simulink model "AER372_lab1"  (R2021b)
settings: Solver=VariableStepAuto  StartTime=0.0  StopTime=10.0  RelTol=1e-3
settings Model: Creator=Emma  LastModifiedBy=Emma

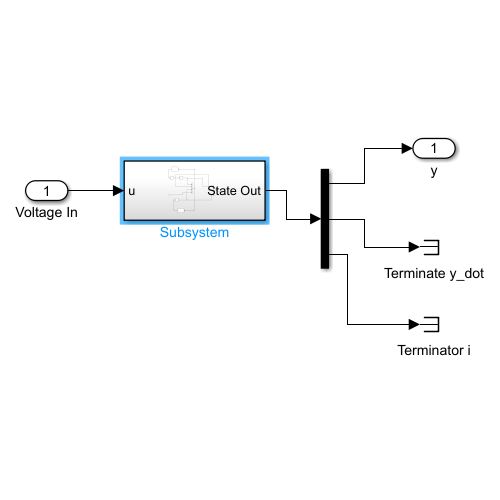
[thumbnail: Simulink's stored preview of the top-level diagram]
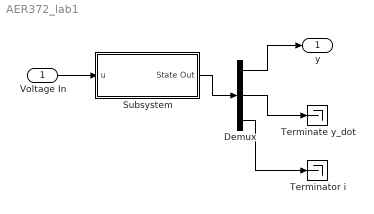
== system AER372_lab1 ==
  Voltage In : Inport
  Demux : Demux  Outputs=3
  Subsystem : Subsystem
  Terminate y_dot : Terminator
  Terminator i : Terminator
  y : Outport
  wires:
  Voltage In/1 -> Subsystem/1(u)
  Demux/1 -> y/1
  Demux/2 -> Terminate y_dot/1
  Demux/3 -> Terminator i/1
  Subsystem/1(State Out) -> Demux/1

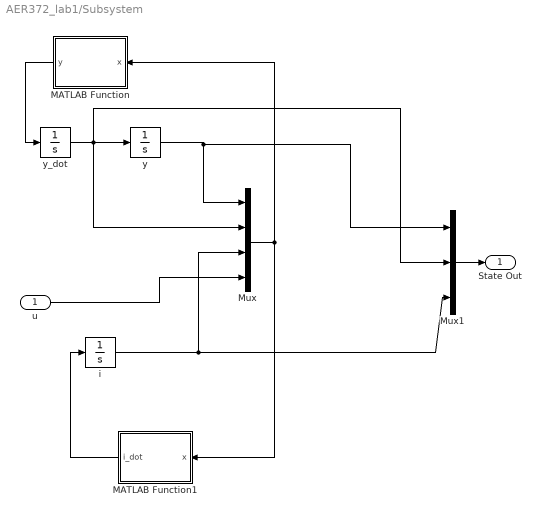
== system AER372_lab1/Subsystem ==
  u : Inport
  MATLAB Function : MATLAB Function  TreatAsAtomicUnit=on
  MATLAB Function1 : MATLAB Function  TreatAsAtomicUnit=on
  Mux : Mux
  Mux1 : Mux  Inputs=3
  i : Integrator
  y : Integrator
  y_dot : Integrator
  State Out : Outport
  wires:
  u/1 -> Mux/4
  Mux1/1 -> State Out/1
  i/1 -> Mux/3, Mux1/3
  y/1 -> Mux1/1, Mux/1
  y_dot/1 -> Mux/2, Mux1/2, y/1
  Mux/1 -> MATLAB Function1/1(x), MATLAB Function/1(x)
  MATLAB Function1/1(i_dot) -> i/1
  MATLAB Function/1(y) -> y_dot/1

== matlab function AER372_lab1/Subsystem/MATLAB Function ==
  data: x input; y output
function y = fcn(x)

y0 = 1;
g = 9.8;
m = 1;
R = 3;
L = 1;

y = x(3)^2/(m*(x(1))^2) - g;

== matlab function AER372_lab1/Subsystem/MATLAB Function1 ==
  data: x input; i_dot output
function i_dot = fcn(x)

y0 = 1;
g = 9.8;
m = 1;
R = 3;
L = 1;

i_dot = x(4)/L -x(3)*R/L;
